simulink model "sampleModel1794"  (R2023a)
settings: Solver=VariableStepAuto  StartTime=0.0  StopTime=10.0  RelTol=1e-3
libraries: hdlsllib x9, simulink x1
settings Model: Creator=user1  LastModifiedBy=user1

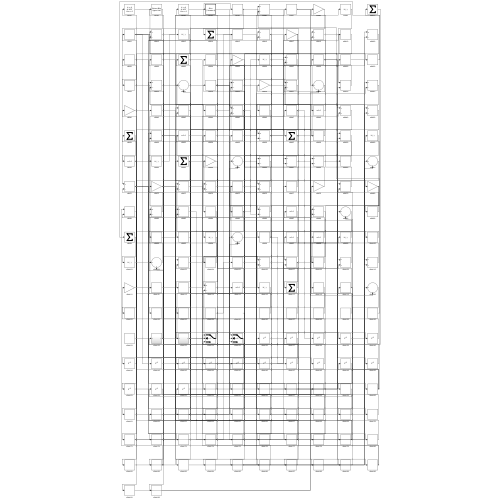
[thumbnail: Simulink's stored preview of the top-level diagram]
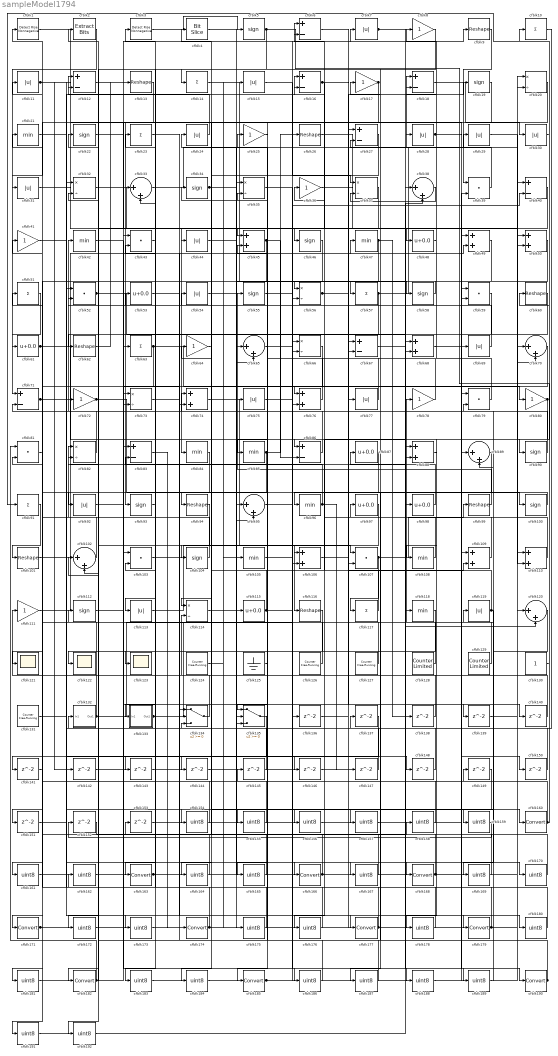
== system sampleModel1794 ==
  cfblk1 : hdlsllib/Logic and Bit Operations/Detect Rise Nonnegative  vinit=0  OutDataTypeStr=boolean
  cfblk{10,14,23,51,57,63,91,117} (8 alike) : Sum  Inputs=+
  cfblk{5,19,22,34,46,55,58,90,93,100,104,112} (12 alike) : Signum
  cfblk{9,13,26,60,62,94,99,101,116} (9 alike) : Reshape
  cfblk{33,38,65,70,89,95,102,120} (8 alike) : Sum  Inputs=|++
  cfblk{39,43,52,59,79,81,103,107} (8 alike) : DotProduct  OutDataTypeStr=Inherit: Inherit via internal rule
  cfblk{21,42,47,84..85,96,105,108,118} (9 alike) : MinMax
  cfblk{45,49..50,68,74,76,88,106,109..110} (10 alike) : Sum
  cfblk{7,11,15,24,28..31,44,54,69,75,77,92,113,119} (16 alike) : Abs  SaturateOnIntegerOverflow=off
  cfblk{8,17,25,36,41,64,72,78,80,111} (10 alike) : Gain
  cfblk{20,32,35,37,56,66,73,82,114} (9 alike) : Product  Inputs=*/  RndMeth=Zero  SaturateOnIntegerOverflow=on
  cfblk{48,53,61,87,97..98,115} (7 alike) : Bias  Bias=0.0  SaturateOnIntegerOverflow=off
  cfblk{6,12,16,18,27,40,67,71,83,86} (10 alike) : Sum  Inputs=+-
  cfblk121 : Scope
  cfblk122 : Scope
  cfblk123 : Scope
  cfblk{124,126..127,131} (4 alike) : hdlsllib/Sources/Counter Free-Running  NumBits=16  tsamp=-1
  cfblk125 : Ground
  cfblk128 : hdlsllib/Sources/Counter Limited  uplimit=7  tsamp=-1
  cfblk129 : hdlsllib/Sources/Counter Limited  uplimit=7  tsamp=-1
  cfblk130 : Constant  SampleTime=-1
  cfblk132 : Subsystem
      settings: LibrarySourceBlock=|
      | hdlsllib/Ports &
      | Subsystems/Subsystem
  cfblk133 : Subsystem
      settings: LibrarySourceBlock=|
      | hdlsllib/Ports &
      | Subsystems/Subsystem
  cfblk134 : Switch  SaturateOnIntegerOverflow=off  InputSameDT=off
  cfblk135 : Switch  SaturateOnIntegerOverflow=off  InputSameDT=off
  cfblk{136..153} (18 alike) : Delay  SampleTime=1
  cfblk{154..159,161..162,164..165,167,169..170,172..173,175..176,178,180..181,183..184,186..189,191..192} (28 alike) : DataTypeConversion  OutDataTypeStr=uint8  SaturateOnIntegerOverflow=off  RndMeth=Floor
  cfblk{160,163,166,168,171,174,177,179,182,185,190} (11 alike) : DataTypeConversion  SaturateOnIntegerOverflow=off  RndMeth=Floor
  cfblk2 : simulink/Logic and Bit Operations/Extract Bits  bitsToExtract=Upper half  numBits=8  bitIdxRange=[0 7]  outScalingMode=Preserve fixed-point scaling
      settings: LibrarySourceBlock=|
      | hdlsllib/Logic and Bit
      | Operations/Extract Bits
  cfblk3 : hdlsllib/Logic and Bit Operations/Detect Rise Nonnegative  vinit=0  OutDataTypeStr=boolean
  cfblk4 : hdlsllib/Logic and Bit Operations/Bit Slice  lidx=7  ridx=0
  wires:
  cfblk2/1 -> cfblk71/1
  cfblk17/1 -> cfblk93/1, cfblk85/1
  cfblk9/1 -> cfblk39/1
  cfblk124/1 -> cfblk105/1
  cfblk98/1 -> cfblk14/1
  cfblk107/1 -> cfblk99/1, cfblk117/1
  cfblk14/1 -> cfblk57/1
  cfblk62/1 -> cfblk13/1
  cfblk100/1 -> cfblk96/1
  cfblk46/1 -> cfblk113/1
  cfblk134/1 -> cfblk111/1
  cfblk113/1 -> cfblk107/1
  cfblk71/1 -> cfblk72/1, cfblk146/1, cfblk148/1
  cfblk76/1 -> cfblk24/1
  cfblk72/1 -> cfblk100/1, cfblk135/3
  cfblk91/1 -> cfblk101/1
  cfblk74/1 -> cfblk116/1
  cfblk3/1 -> cfblk5/1
  cfblk58/1 -> cfblk56/1
  cfblk63/1 -> cfblk80/1, cfblk151/1
  cfblk81/1 -> cfblk121/1
  cfblk5/1 -> cfblk90/1, cfblk133/1(In1)
  cfblk18/1 -> cfblk30/1
  cfblk33/1 -> cfblk18/1
  cfblk1/1 -> cfblk45/1
  cfblk35/1 -> cfblk168/1
  cfblk111/1 -> cfblk47/1
  cfblk108/1 -> cfblk17/1
  cfblk20/1 -> cfblk114/1
  cfblk85/1 -> cfblk26/1, cfblk191/1
  cfblk129/1 -> cfblk78/1
  cfblk36/1 -> cfblk98/1
  cfblk43/1 -> cfblk163/1
  cfblk24/1 -> cfblk12/1
  cfblk10/1 -> cfblk132/1(In1)
  cfblk29/1 -> cfblk110/1
  cfblk19/1 -> cfblk135/1
  cfblk90/1 -> cfblk55/1
  cfblk55/1 -> cfblk7/1
  cfblk44/1 -> cfblk28/1
  cfblk25/1 -> cfblk185/1
  cfblk77/1 -> cfblk34/1
  cfblk82/1 -> cfblk42/1
  cfblk51/1 -> cfblk61/1
  cfblk83/1 -> cfblk174/1
  cfblk31/1 -> cfblk109/1
  cfblk78/1 -> cfblk16/1
  cfblk26/1 -> cfblk110/2
  cfblk41/1 -> cfblk16/2
  cfblk57/1 -> cfblk20/1, cfblk172/1
  cfblk15/1 -> cfblk37/1
  cfblk61/1 -> cfblk86/1, cfblk161/1
  cfblk103/1 -> cfblk106/1
  cfblk116/1 -> cfblk122/1
  cfblk50/1 -> cfblk171/1
  cfblk119/1 -> cfblk36/1, cfblk159/1
  cfblk79/1 -> cfblk18/2
  cfblk92/1 -> cfblk9/1
  cfblk38/1 -> cfblk37/2
  cfblk101/1 -> cfblk88/1
  cfblk66/1 -> cfblk76/1
  cfblk106/1 -> cfblk109/2
  cfblk132/1(Out1) -> cfblk65/1, cfblk81/2
  cfblk130/1 -> cfblk60/1
  cfblk39/1 -> cfblk27/2
  cfblk47/1 -> cfblk66/2, cfblk138/1
  cfblk32/1 -> cfblk84/1
  cfblk115/1 -> cfblk64/1, cfblk40/2
  cfblk73/1 -> cfblk179/1
  cfblk102/1 -> cfblk82/1
  cfblk11/1 -> cfblk49/1, cfblk33/1, cfblk142/1, cfblk170/1
  cfblk54/1 -> cfblk135/2
  cfblk30/1 -> cfblk91/1
  cfblk109/1 -> cfblk87/1
  cfblk68/1 -> cfblk190/1
  cfblk70/1 -> cfblk182/1
  cfblk127/1 -> cfblk3/1
  cfblk64/1 -> cfblk94/1
  cfblk48/1 -> cfblk8/1
  cfblk60/1 -> cfblk106/2
  cfblk52/1 -> cfblk118/1, cfblk74/2
  cfblk12/1 -> cfblk6/1
  cfblk16/1 -> cfblk46/1, cfblk48/1
  cfblk86/1 -> cfblk41/1
  cfblk21/1 -> cfblk177/1
  cfblk133/1(Out1) -> cfblk76/2, cfblk49/2
  cfblk45/1 -> cfblk92/1, cfblk86/2
  cfblk34/1 -> cfblk115/1, cfblk29/1, cfblk88/2
  cfblk6/1 -> cfblk67/2
  cfblk117/1 -> cfblk4/1
  cfblk96/1 -> cfblk33/2, cfblk147/1
  cfblk8/1 -> cfblk62/1
  cfblk104/1 -> cfblk51/1
  cfblk80/1 -> cfblk108/1, cfblk176/1
  cfblk7/1 -> cfblk38/1, cfblk120/2
  cfblk56/1 -> cfblk19/1, cfblk140/1
  cfblk128/1 -> cfblk2/1
  cfblk4/1 -> cfblk58/1
  cfblk93/1 -> cfblk123/1
  cfblk126/1 -> cfblk74/1
  cfblk94/1 -> cfblk102/2
  cfblk69/1 -> cfblk32/2
  cfblk110/1 -> cfblk6/2
  cfblk99/1 -> cfblk75/1
  cfblk13/1 -> cfblk31/1
  cfblk112/1 -> cfblk166/1
  cfblk22/1 -> cfblk44/1
  cfblk37/1 -> cfblk56/2
  cfblk28/1 -> cfblk69/1, cfblk150/1
  cfblk95/1 -> cfblk160/1
  cfblk27/1 -> cfblk104/1
  cfblk136/1 -> cfblk107/2
  cfblk138/1 -> cfblk102/1
  cfblk23/1 -> cfblk139/1
  cfblk139/1 -> cfblk20/2
  cfblk140/1 -> cfblk114/2
  cfblk135/1 -> cfblk141/1
  cfblk141/1 -> cfblk1/1
  cfblk142/1 -> cfblk66/1
  cfblk49/1 -> cfblk143/1
  cfblk143/1 -> cfblk65/2
  cfblk118/1 -> cfblk144/1
  cfblk144/1 -> cfblk67/1
  cfblk145/1 -> cfblk134/2
  cfblk146/1 -> cfblk27/1
  cfblk147/1 -> cfblk32/1
  cfblk148/1 -> cfblk82/2
  cfblk150/1 -> cfblk134/3
  cfblk153/1 -> cfblk39/2
  cfblk131/1 -> cfblk154/1
  cfblk154/1 -> cfblk53/1
  cfblk59/1 -> cfblk155/1
  cfblk155/1 -> cfblk71/2
  cfblk87/1 -> cfblk156/1
  cfblk156/1 -> cfblk59/1
  cfblk53/1 -> cfblk157/1
  cfblk157/1 -> cfblk59/2
  cfblk152/1 -> cfblk158/1
  cfblk158/1 -> cfblk45/2
  cfblk159/1 -> cfblk152/1
  cfblk160/1 -> cfblk149/1, cfblk52/2, cfblk79/2, cfblk10/1
  cfblk161/1 -> cfblk95/1
  cfblk162/1 -> cfblk95/2
  cfblk163/1 -> cfblk38/2, cfblk23/1
  cfblk97/1 -> cfblk164/1
  cfblk164/1 -> cfblk43/1
  cfblk125/1 -> cfblk165/1
  cfblk165/1 -> cfblk43/2
  cfblk166/1 -> cfblk103/2, cfblk120/1, cfblk11/1
  cfblk65/1 -> cfblk167/1
  cfblk167/1 -> cfblk112/1
  cfblk168/1 -> cfblk54/1, cfblk97/1
  cfblk120/1 -> cfblk169/1
  cfblk169/1 -> cfblk35/1
  cfblk170/1 -> cfblk35/2
  cfblk171/1 -> cfblk103/1, cfblk63/1
  cfblk172/1 -> cfblk50/1
  cfblk151/1 -> cfblk173/1
  cfblk173/1 -> cfblk50/2
  cfblk174/1 -> cfblk12/2, cfblk15/1, cfblk77/1
  cfblk114/1 -> cfblk175/1
  cfblk175/1 -> cfblk83/1
  cfblk176/1 -> cfblk83/2
  cfblk177/1 -> cfblk145/1, cfblk52/1
  cfblk88/1 -> cfblk178/1
  cfblk178/1 -> cfblk21/1
  cfblk179/1 -> cfblk153/1, cfblk79/1, cfblk119/1
  cfblk75/1 -> cfblk180/1
  cfblk180/1 -> cfblk73/1
  cfblk137/1 -> cfblk181/1
  cfblk181/1 -> cfblk73/2
  cfblk182/1 -> cfblk162/1, cfblk81/1
  cfblk84/1 -> cfblk183/1
  cfblk183/1 -> cfblk70/1
  cfblk149/1 -> cfblk184/1
  cfblk184/1 -> cfblk70/2
  cfblk185/1 -> cfblk136/1, cfblk40/1
  cfblk42/1 -> cfblk186/1
  cfblk186/1 -> cfblk25/1
  cfblk89/1 -> cfblk187/1
  cfblk187/1 -> cfblk22/1
  cfblk105/1 -> cfblk188/1
  cfblk188/1 -> cfblk89/1
  cfblk67/1 -> cfblk189/1
  cfblk189/1 -> cfblk89/2
  cfblk190/1 -> cfblk137/1, cfblk134/1
  cfblk191/1 -> cfblk68/1
  cfblk40/1 -> cfblk192/1
  cfblk192/1 -> cfblk68/2

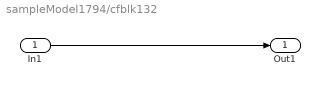
== system sampleModel1794/cfblk132 ==
  In1 : Inport
  Out1 : Outport
  wires:
  In1/1 -> Out1/1

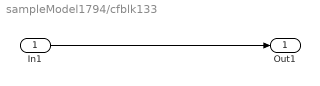
== system sampleModel1794/cfblk133 ==
  In1 : Inport
  Out1 : Outport
  wires:
  In1/1 -> Out1/1
